simulink model "vending_machine"  (R2020b)
settings: Solver=VariableStepAuto  StartTime=0.0  StopTime=200  RelTol=1e-3
settings Model: Creator=sayali  LastModifiedBy=sayali

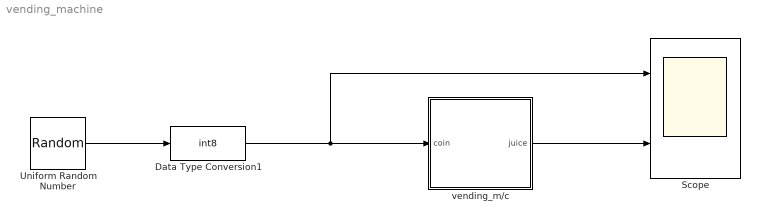
== system vending_machine ==
  Data Type Conversion1 : DataTypeConversion  OutDataTypeStr=int8  RndMeth=Nearest  SaturateOnIntegerOverflow=on
  Scope : Scope  NumInputPorts=2
  Uniform Random Number : UniformRandomNumber  Minimum=0  Maximum=2  Seed=337  SampleTime=10
  vending_m/c : Stateflow chart  TreatAsAtomicUnit=on
  wires:
  Uniform Random Number/1 -> Data Type Conversion1/1
  Data Type Conversion1/1 -> Scope/1, vending_m/c/1(coin)
  vending_m/c/1(juice) -> Scope/2

== stateflow chart vending_machine/vending_m//c ==
  state got_0
  state got_dime
  state got_nickel
  (default) -> got_0
  got_0 -> got_dime [order 2] : [coin==2]{juice=0}
  got_dime -> got_0 [order 1] : [coin==1]{juice=1}
  got_0 -> got_nickel [order 1] : [coin==1]{juice=0}
  got_nickel -> got_0 [order 2] : [coin==2]{juice=1}
  got_nickel -> got_dime [order 1] : [coin==1]{juice=0}
  got_dime -> got_nickel [order 2] : [coin==2]{juice=1}
  data: coin input; juice output
